simulink model "HVDC_VSC_1CPUcore_dcpl"  (Simulink 8.4)
settings: Solver=ode3  SolverMode=SingleTasking  StartTime=0.0  StopTime=70.0  FixedStep=Ts_Power  RelTol=1e-3  AbsTol=1e-2
PreLoadFcn:
  | Ts_Power=50e-6; Ts_Control=1*Ts_Power; init_cosim_IA; startup_transients_hvdc_vsc;
PostLoadFcn:
  | Ts_Power=50e-6; Ts_Control=1*Ts_Power; init_cosim_IA; startup_transients_hvdc_vsc;
InitFcn:
  | Ts_Power=50e-6; Ts_Control=1*Ts_Power; init_cosim_IA; startup_transients_hvdc_vsc;
values from neighbouring files (symbols this model uses):
  dPref1_2 = 0.125    [startup_transients_hvdc_vsc.m]
  dPref1_2_rlimit = 0.6    [startup_transients_hvdc_vsc.m]
  t_deblock_Pref1 = 0.5    [startup_transients_hvdc_vsc.m]
  t_deblock_Udref2 = 0.3    [startup_transients_hvdc_vsc.m]
  t_dPref1_2 = 25.0    (= 25)    [startup_transients_hvdc_vsc.m]
  t_SwitchITMIdc = 0.2    [startup_transients_hvdc_vsc.m]
  t_SwitchITMVdc = 0.1    [startup_transients_hvdc_vsc.m]
undefined symbols (not defined in the file or in its folder): CLARK, D1, Delta, gcbh, h, intfDelay, level, lib_mesures, magnitude, ResistanceM, rte_drive_private_lib, rte_tsb3level_hiz_rect_cb, sps_rtmsupport, Ts_intf, TSB3_hiZR
libraries: powerlib x183, spsVIMeasurementModel x102, powerlib_extras x71, powerlib_meascontrol x50, rteventslib x26, op_dpl_lib x20, rtlab x12, sps_avr x6, artemis x1
(part 9 of 13)

== system HVDC_VSC_1CPUcore_dcpl/SM_HVDC_VSC/VSC Controller (Station 1)/3-level firing pulse unit for TSB/Subsystem2 ==
  in : Inport
  c+ : Inport  Port=2
  c- : Inport  Port=3
  RTE Logical Operator : rteventslib/Math Operations/RTE Logical Operator  LogicalOperator=NOT  NbrInput=1  NbrMaxEvents=1
  RTE Logical Operator1 : rteventslib/Math Operations/RTE Logical Operator  LogicalOperator=NOT  NbrInput=1  NbrMaxEvents=1
  RTE Relational Operator2 : rteventslib/Math Operations/RTE Relational Operator  RelationalOperator=>=  NumberMaxEvents=1  SampleTime=Ts
  RTE Relational Operator3 : rteventslib/Math Operations/RTE Relational Operator  RelationalOperator=<=  NumberMaxEvents=1  SampleTime=Ts
  1 : Outport
  2 : Outport  Port=2
  3 : Outport  Port=3
  4 : Outport  Port=4
  wires:
  RTE Logical Operator/1 -> 3/1
  RTE Logical Operator1/1 -> 2/1
  RTE Relational Operator3/1 -> 4/1, RTE Logical Operator1/1
  RTE Relational Operator2/1 -> 1/1, RTE Logical Operator/1
  c-/1 -> RTE Relational Operator3/2
  c+/1 -> RTE Relational Operator2/2
  in/1 -> RTE Relational Operator2/1, RTE Relational Operator3/1

== system HVDC_VSC_1CPUcore_dcpl/SM_HVDC_VSC/VSC Controller (Station 1)/3-level firing pulse unit for TSB/Subsystem6 ==
  in : Inport
  c+ : Inport  Port=2
  c- : Inport  Port=3
  RTE Logical Operator : rteventslib/Math Operations/RTE Logical Operator  LogicalOperator=NOT  NbrInput=1  NbrMaxEvents=1
  RTE Logical Operator1 : rteventslib/Math Operations/RTE Logical Operator  LogicalOperator=NOT  NbrInput=1  NbrMaxEvents=1
  RTE Relational Operator2 : rteventslib/Math Operations/RTE Relational Operator  RelationalOperator=>=  NumberMaxEvents=1  SampleTime=Ts
  RTE Relational Operator3 : rteventslib/Math Operations/RTE Relational Operator  RelationalOperator=<=  NumberMaxEvents=1  SampleTime=Ts
  1 : Outport
  2 : Outport  Port=2
  3 : Outport  Port=3
  4 : Outport  Port=4
  wires:
  RTE Logical Operator/1 -> 3/1
  RTE Logical Operator1/1 -> 2/1
  RTE Relational Operator3/1 -> 4/1, RTE Logical Operator1/1
  RTE Relational Operator2/1 -> 1/1, RTE Logical Operator/1
  c-/1 -> RTE Relational Operator3/2
  c+/1 -> RTE Relational Operator2/2
  in/1 -> RTE Relational Operator2/1, RTE Relational Operator3/1

== system HVDC_VSC_1CPUcore_dcpl/SM_HVDC_VSC/VSC Controller (Station 1)/Discrete VSC Controller (Station 1)/Clark Transformations ==
  note: 0: Y-Y
      | 1: Y-D1
      | 2: Y-D11
  note: Clark's Transformations
  "U_abc " : Inport
  "I_abc " : Inport  Port=2
  "Uf_abc " : Inport  Port=3
  "Iv_abc " : Inport  Port=4
  "CLARK " : Subsystem  AncestorBlock=lib_mesures/CLARK
  "CLARK  " : Subsystem  AncestorBlock=lib_mesures/CLARK
  CLARK_YD : Subsystem
  "CLARK_YD " : Subsystem
  Constant2 : Constant  Value=Tr_connection
  Selector{,1..3} (4 alike) : Selector  InputPortWidth=3  Indices=[1 2]
  U_AB : Outport
  I_AB : Outport  Port=2
  Uf_AB : Outport  Port=3
  Iv_AB : Outport  Port=4
  wires:
  Constant2/1 -> "CLARK_YD "/2(Tr_conx), CLARK_YD/2(Tr_conx)
  "U_abc "/1 -> CLARK_YD/1(abc)
  "I_abc "/1 -> "CLARK_YD "/1(abc)
  "Uf_abc "/1 -> "CLARK "/1(abc)
  "Iv_abc "/1 -> "CLARK  "/1(abc)
  CLARK_YD/1(AB0) -> Selector/1
  "CLARK "/1(AB0) -> Selector2/1
  "CLARK  "/1(AB0) -> Selector3/1
  "CLARK_YD "/1(AB0) -> Selector1/1
  Selector/1 -> U_AB/1
  Selector1/1 -> I_AB/1
  Selector2/1 -> Uf_AB/1
  Selector3/1 -> Iv_AB/1

== system HVDC_VSC_1CPUcore_dcpl/SM_HVDC_VSC/VSC Controller (Station 1)/Discrete VSC Controller (Station 1)/DC Voltage Balance Control ==
  note: DC Voltage Balance Control
  Vref_lim_abc : Inport
  Iv_abc : Inport  Port=2
  Udc_pn : Inport  Port=3
  Freq : Inport  Port=4
  activate_reg : Inport  Port=5
  Constant8 : Constant  Value=0
  First-Order_LP f0_dcvbc : powerlib_extras/Discrete  Control Blocks/Discrete 1st-Order Filter  FilterType=Lowpass  Tc=1/(2*pi*f0_dcvbc)  Ts=Ts_Control  Initialize=off  Vac_Init=[0.8 -25 60]  Vdc_Init=-0.4  PlotResponse=off  param1=[1 500 0.1]
  Gain4 : Gain  Gain=k_pu2nom_Vdc  SaturateOnIntegerOverflow=on  OutDataTypeStr=Inherit: Same as input  ParamDataTypeStr=Inherit: Same as input
  Regulator : Subsystem  TreatAsAtomicUnit=on
  Sum : Sum  Inputs=1  SaturateOnIntegerOverflow=on
  Switch2 : Switch  Threshold=0.5  SaturateOnIntegerOverflow=on
  Variable Frequency Mean value : powerlib_extras/Discrete Measurements/Discrete Variable Frequency Mean value  Finit=60  Fmin=f_min_pll  Vinit=0  Ts=Ts_Control
  dVref_abc : Outport
  Udc_0_mean : Outport  Port=2
  wires:
  First-Order_LP f0_dcvbc/1 -> Variable Frequency Mean value/2
  Sum/1 -> First-Order_LP f0_dcvbc/1
  Vref_lim_abc/1 -> Regulator/1(V_ref_lim_abc)
  Iv_abc/1 -> Regulator/2(Iv_abc)
  Udc_pn/1 -> Sum/1
  Freq/1 -> Variable Frequency Mean value/1
  Variable Frequency Mean value/1 -> Gain4/1
  Gain4/1 -> Regulator/3(Udc_0_mean), Udc_0_mean/1
  Regulator/1(dV_ref_abc_dcvbc) -> Switch2/1
  Switch2/1 -> dVref_abc/1
  Constant8/1 -> Switch2/3
  activate_reg/1 -> Regulator/Enable, Switch2/2

== system HVDC_VSC_1CPUcore_dcpl/SM_HVDC_VSC/VSC Controller (Station 1)/Discrete VSC Controller (Station 1)/Inner Current Loop ==
  note: Inner Current Loop
  U_dq : Inport
  Iv_dq : Inport  Port=2
  Udc_meas : Inport  Port=3
  Iref_dq : Inport  Port=4
  Freq : Inport  Port=5
  sin_cos : Inport  Port=6
  AC_Current_Control : Subsystem
  Constant1 : Constant  Value=0
  Inverse_Clark : Subsystem  AncestorBlock=lib_mesures/CLARK
  Max=10 Min=0 : Saturate  UpperLimit=10  LowerLimit=0
  Mux1 : Mux  Inputs=[2 1]
  Reference_Voltage_Conditioning : Subsystem
  Reference_Voltage_Limitation : Subsystem
  Selector : Selector  InputPortWidth=3  Indices=[ 1 2]
  Variable Frequency Mean value IC:1.0 : powerlib_extras/Discrete Measurements/Discrete Variable Frequency Mean value  Finit=60  Fmin=f_min_pll  Vinit=1.0  Ts=Ts_Control
  dq0 to abo : Subsystem  AncestorBlock=lib_mesures/CLARK
  Vref_lim_abc : Outport
  Vref_lim_AB : Outport  Port=2
  wires:
  Selector/1 -> Vref_lim_AB/1
  Reference_Voltage_Limitation/1(Vref_lim_dq) -> Mux1/1
  Inverse_Clark/1(abc) -> Vref_lim_abc/1
  Mux1/1 -> dq0 to abo/1(dq0)
  Constant1/1 -> Mux1/2
  sin_cos/1 -> dq0 to abo/2(sin_cos)
  dq0 to abo/1(ab0) -> Selector/1, Inverse_Clark/1(AB0)
  Udc_meas/1 -> Variable Frequency Mean value IC:1.0/2
  Variable Frequency Mean value IC:1.0/1 -> Max=10 Min=0/1
  Freq/1 -> Variable Frequency Mean value IC:1.0/1, AC_Current_Control/4(Freq)
  Iref_dq/1 -> AC_Current_Control/2(Iref_dq)
  U_dq/1 -> AC_Current_Control/3(U_dq)
  Reference_Voltage_Conditioning/1(Vref_dq) -> Reference_Voltage_Limitation/1(Vref_dq)
  AC_Current_Control/1(Vref_dq_tmp) -> Reference_Voltage_Conditioning/1(Vref_dq_tmp)
  Max=10 Min=0/1 -> Reference_Voltage_Conditioning/2(Udc_meas_mean)
  Iv_dq/1 -> AC_Current_Control/1(Iv_dq)

== system HVDC_VSC_1CPUcore_dcpl/SM_HVDC_VSC/VSC Controller (Station 1)/Discrete VSC Controller (Station 1)/Outer Active-Reactive Power and Voltage Loop ==
  note: Outer Active-Reactive Power and Voltage Loop
  Udc_meas : Inport
  Uf_meas : Inport  Port=2
  P_meas : Inport  Port=3
  Q_meas : Inport  Port=4
  U_meas : Inport  Port=5
  Pref : Inport  Port=6
  dPref : Inport  Port=7
  Qref : Inport  Port=8
  Udref : Inport  Port=9
  block_status : Inport  Port=10
  Active_Power_Control : Subsystem
  Constant19 : Constant  Value=Ki_dcvc
  Constant20 : Constant  Value=Kp_dcvc
  Constant9 : Constant  Value=P_control
  Current_Reference_Calculation : Subsystem
  Current_Reference_Limitation : Subsystem
  DC_Voltage_Control : Subsystem  TreatAsAtomicUnit=on
  Logical Operator1 : Logic  AllPortsSameDT=off
  Logical Operator4 : Logic  Operator=NOT  AllPortsSameDT=off
  Logical Operator6 : Logic  AllPortsSameDT=off
  Logical Operator7 : Logic  Operator=NOT  AllPortsSameDT=off
  Reactive_Power_Control : Subsystem
  Switch2 : Switch  Threshold=0.5  SaturateOnIntegerOverflow=on
  Iref_dq : Outport
  Pref_ramped : Outport  Port=2
  wires:
  Current_Reference_Limitation/1(Iref_dq) -> Iref_dq/1
  Switch2/1 -> Current_Reference_Limitation/1(Iref_d_tmp)
  Logical Operator4/1 -> Logical Operator1/1, Logical Operator6/2, Active_Power_Control/2(enable_ramp), Reactive_Power_Control/1(enable_control)
  Current_Reference_Calculation/1(Iref_d_crc) -> Switch2/1
  Constant20/1 -> DC_Voltage_Control/4(Kp_dcvc)
  Constant19/1 -> DC_Voltage_Control/3(Ki_dcvc)
  Q_meas/1 -> Reactive_Power_Control/3(Q_meas)
  P_meas/1 -> Active_Power_Control/5(P_meas)
  DC_Voltage_Control/1(Iref_d_dcvc) -> Switch2/3
  Udc_meas/1 -> Active_Power_Control/7(Udc_meas), DC_Voltage_Control/2(Udc_meas)
  block_status/1 -> Logical Operator4/1
  Constant9/1 -> Logical Operator6/1, Current_Reference_Limitation/3(P_control), Logical Operator7/1
  Logical Operator6/1 -> Switch2/2, Active_Power_Control/1(enable_control)
  U_meas/1 -> Reactive_Power_Control/4(U_meas), Active_Power_Control/6(U_meas)
  Current_Reference_Calculation/2(Iref_q_crc) -> Current_Reference_Limitation/2(Iref_q_tmp)
  dPref/1 -> Active_Power_Control/4(dPref)
  Active_Power_Control/1(Pref_apc) -> Current_Reference_Calculation/1(Pref_apc)
  Reactive_Power_Control/1(Qref_rpc) -> Current_Reference_Calculation/2(Qref_rpc)
  Pref/1 -> Active_Power_Control/3(Pref)
  Uf_meas/1 -> Current_Reference_Calculation/3(Uf_meas)
  Qref/1 -> Reactive_Power_Control/2(Qref)
  Logical Operator7/1 -> Logical Operator1/2
  Logical Operator1/1 -> DC_Voltage_Control/Enable
  Udref/1 -> DC_Voltage_Control/1(Udref)
  Active_Power_Control/2(Pref_ramped) -> Pref_ramped/1

== system HVDC_VSC_1CPUcore_dcpl/SM_HVDC_VSC/VSC Controller (Station 1)/Discrete VSC Controller (Station 1)/PLL ==
  note: Discrete 3-phase PLL
  note: Pierre Giroux, Gilbert Sybille
      | Power System Laboratory, IREQ
      | Hydro-Quebec
  U_AB : Inport
  Constant1 : Constant  Value=0
  Constant4 : Constant  Value=2*pi
  Discrete PI Controller : powerlib_extras/Discrete  Control Blocks/Discrete PI Controller  Kp=Kp  Ki=Ki  Par_Limits=2*pi*Finit*[1.25 0.75]  Init=2*pi*Finit  Ts=Ts
  Discrete Rate Limiter : powerlib_extras/Discrete  Control Blocks/Discrete Rate Limiter  R=12  F=-12  Vinit=Finit  Ts=Ts
  Discrete Variable Frequency Mean value : powerlib_extras/Discrete Measurements/Discrete Variable Frequency Mean value  Finit=Finit  Fmin=Fmin  Vinit=0  Ts=Ts
  Discrete  2nd-Order Filter : powerlib_extras/Discrete  Control Blocks/Discrete  2nd-Order Filter  FilterType=Lowpass  Fo=30  Zeta=0.707  Ts=Ts  Initialize=on  Vac_Init=[0 0 Finit]  Vdc_Init=Finit  PlotResponse=off  param1=[1 500 0.1]
  Discrete-Time Integrator : DiscreteIntegrator  InitialCondition=Phase_Init*pi/180  SampleTime=Ts
  Gain10 : Gain  Gain=1/2/pi  SaturateOnIntegerOverflow=on  OutDataTypeStr=Inherit: Same as input  ParamDataTypeStr=Inherit: Same as input
  Math Function : Math  Operator=mod  SaturateOnIntegerOverflow=on
  Mux1 : Mux  Inputs=[2 1]
  Mux2 : Mux  Inputs=2
  Selector : Selector  InputPortWidth=3  Indices=2
  Trigonometric Function : Trigonometry
  Trigonometric Function2 : Trigonometry  Operator=cos
  Unit Delay : UnitDelay  InitialCondition=Finit  SampleTime=Ts
  "ab0->dq0 " : Subsystem  AncestorBlock=lib_mesures/CLARK
  Freq : Outport
  theta : Outport  Port=2
  Sin_Cos : Outport  Port=3
  wires:
  Constant1/1 -> Mux1/2
  Mux1/1 -> "ab0->dq0 "/1(ab0)
  U_AB/1 -> Mux1/1
  Discrete Variable Frequency Mean value/1 -> Discrete PI Controller/1
  "ab0->dq0 "/1(dq0) -> Selector/1
  Constant4/1 -> Math Function/2
  Discrete-Time Integrator/1 -> Math Function/1
  Math Function/1 -> Trigonometric Function/1, Trigonometric Function2/1, theta/1
  Trigonometric Function/1 -> Mux2/1
  Trigonometric Function2/1 -> Mux2/2
  Mux2/1 -> "ab0->dq0 "/2(sin_cos), Sin_Cos/1
  Discrete PI Controller/1 -> Discrete-Time Integrator/1, Gain10/1  "W"
  Gain10/1 -> Discrete Rate Limiter/1
  Discrete Rate Limiter/1 -> Discrete  2nd-Order Filter/1
  Unit Delay/1 -> Freq/1, Discrete Variable Frequency Mean value/1
  Discrete  2nd-Order Filter/1 -> Unit Delay/1
  Selector/1 -> Discrete Variable Frequency Mean value/2  "Vq"

== system HVDC_VSC_1CPUcore_dcpl/SM_HVDC_VSC/VSC Controller (Station 1)/Discrete VSC Controller (Station 1)/Signal Calculations ==
  U_AB : Inport
  I_AB : Inport  Port=2
  Uf_AB : Inport  Port=3
  Vref_lim_AB : Inport  Port=4
  Udc_pn : Inport  Port=5
  Idc_pn : Inport  Port=6
  Freq : Inport  Port=7
  2nd-Order Filter : powerlib_extras/Discrete  Control Blocks/Discrete  2nd-Order Filter  FilterType=Lowpass  Fo=f0_sc  Zeta=zeta_sc  Ts=Ts_Control  Initialize=off  Vac_Init=[0.8 -25 60]  Vdc_Init=-0.4  PlotResponse=off  param1=[1 500 1]
  2nd-Order Filter2 : powerlib_extras/Discrete  Control Blocks/Discrete  2nd-Order Filter  FilterType=Lowpass  Fo=f0_sc  Zeta=zeta_sc  Ts=Ts_Control  Initialize=off  Vac_Init=[0.8 -25 60]  Vdc_Init=-0.4  PlotResponse=off  param1=[1 500 1]
  "2nd-Order Filter " : powerlib_extras/Discrete  Control Blocks/Discrete  2nd-Order Filter  FilterType=Lowpass  Fo=f0_sc  Zeta=zeta_sc  Ts=Ts_Control  Initialize=off  Vac_Init=[0.8 -25 60]  Vdc_Init=-0.4  PlotResponse=off  param1=[1 500 1]
  "2nd-Order Filter  " : powerlib_extras/Discrete  Control Blocks/Discrete  2nd-Order Filter  FilterType=Lowpass  Fo=f0_sc  Zeta=zeta_sc  Ts=Ts_Control  Initialize=off  Vac_Init=[0.8 -25 60]  Vdc_Init=-0.4  PlotResponse=off  param1=[1 500 1]
  2nd-Order Filter 1\ : powerlib_extras/Discrete  Control Blocks/Discrete  2nd-Order Filter  FilterType=Lowpass  Fo=f0_sc  Zeta=zeta_sc  Ts=Ts_Control  Initialize=off  Vac_Init=[0.8 -25 60]  Vdc_Init=-0.4  PlotResponse=off  param1=[1 500 1]
  Active_Power : Subsystem
  DC_Current : Subsystem
  DC_Voltage : Subsystem
  Demux : Demux  Outputs=2
  Demux1 : Demux  Outputs=2
  Filter_Bus_Voltage : Subsystem
  Gain1 : Gain  Gain=k_pu2nom_Vdc*k_pu2nom_Idc  SaturateOnIntegerOverflow=on  OutDataTypeStr=Inherit: Same as input  ParamDataTypeStr=Inherit: Same as input
  Modulation_Index : Subsystem
  PCC_Voltage : Subsystem
  Product5 : Product  SaturateOnIntegerOverflow=on  OutDataTypeStr=Inherit: Same as first input
  Reactive_Power : Subsystem
  Variable Frequency Mean value IC: 0 : powerlib_extras/Discrete Measurements/Discrete Variable Frequency Mean value  Finit=60  Fmin=f_min_pll  Vinit=0  Ts=Ts_Control
  Pdc_meas : Outport
  Mod_index : Outport  Port=2
  Udc_meas : Outport  Port=3
  Uf_meas : Outport  Port=4
  P_meas : Outport  Port=5
  Q_meas : Outport  Port=6
  U_meas : Outport  Port=7
  wires:
  Gain1/1 -> Pdc_meas/1
  Freq/1 -> Variable Frequency Mean value IC: 0/1
  Product5/1 -> Gain1/1
  Variable Frequency Mean value IC: 0/1 -> Product5/2
  2nd-Order Filter 1\/1 -> Uf_meas/1
  "2nd-Order Filter "/1 -> Mod_index/1
  Filter_Bus_Voltage/1(Uf_meas) -> 2nd-Order Filter 1\/1
  PCC_Voltage/1(Upcc) -> "2nd-Order Filter  "/1
  "2nd-Order Filter  "/1 -> U_meas/1
  Active_Power/1(Ppcc) -> 2nd-Order Filter/1
  2nd-Order Filter/1 -> P_meas/1
  Reactive_Power/1(Qpcc) -> 2nd-Order Filter2/1
  2nd-Order Filter2/1 -> Q_meas/1
  Modulation_Index/1(Mod_index) -> "2nd-Order Filter "/1
  Demux/2 -> DC_Voltage/2(Udc_n)
  Uf_AB/1 -> Filter_Bus_Voltage/1(Uf_AB)
  U_AB/1 -> PCC_Voltage/1(U_AB), Active_Power/1(U_AB), Reactive_Power/1(U_AB)
  I_AB/1 -> Active_Power/2(I_AB), Reactive_Power/2(I_AB)
  DC_Voltage/1(Udc_meas) -> Product5/1, Udc_meas/1, Modulation_Index/2(Udc_meas)
  DC_Current/1(Idc_meas) -> Variable Frequency Mean value IC: 0/2
  Udc_pn/1 -> Demux/1
  Demux/1 -> DC_Voltage/1(Udc_p)
  Demux1/1 -> DC_Current/1(Idc_p)
  Demux1/2 -> DC_Current/2(Idc_n)
  Idc_pn/1 -> Demux1/1
  Vref_lim_AB/1 -> Modulation_Index/1(Vref_lim_AB)

== system HVDC_VSC_1CPUcore_dcpl/SM_HVDC_VSC/VSC Controller (Station 1)/Discrete VSC Controller (Station 1)/dq  Transformations ==
  note: dq Transformations
  U_AB : Inport
  Iv_AB : Inport  Port=2
  sin_cos : Inport  Port=3
  Constant1 : Constant  Value=0
  Mux1 : Mux  Inputs=[2 1]
  Mux4 : Mux  Inputs=[2 1]
  Selector : Selector  InputPortWidth=3  Indices=[1 2]
  Selector3 : Selector  InputPortWidth=3  Indices=[1 2]
  ab0_to_dq0 : Subsystem  AncestorBlock=lib_mesures/CLARK
  "ab0_to_dq0   " : Subsystem  AncestorBlock=lib_mesures/CLARK
  U_dq : Outport
  Iv_dq : Outport  Port=2
  wires:
  Constant1/1 -> Mux4/2, Mux1/2
  Mux4/1 -> "ab0_to_dq0   "/1(ab0)
  Iv_AB/1 -> Mux4/1
  Mux1/1 -> ab0_to_dq0/1(ab0)
  U_AB/1 -> Mux1/1
  "ab0_to_dq0   "/1(dq0) -> Selector3/1
  ab0_to_dq0/1(dq0) -> Selector/1
  sin_cos/1 -> "ab0_to_dq0   "/2(sin_cos), ab0_to_dq0/2(sin_cos)
  Selector/1 -> U_dq/1
  Selector3/1 -> Iv_dq/1

== system HVDC_VSC_1CPUcore_dcpl/SM_HVDC_VSC/VSC Controller (Station 2)/3-level firing pulse unit for TSB/Carriers Generator ==
  theta : Inport
  Constant2 : Constant  Value=0.5
  Gain1 : Gain  Gain=1/pi  SaturateOnIntegerOverflow=on  OutDataTypeStr=Inherit: Same as input  ParamDataTypeStr=Inherit: Same as input
  Sum1 : Sum  SaturateOnIntegerOverflow=on  InputSameDT=on  OutDataTypeStr=Inherit: Same as first input
  Sum2 : Sum  Inputs=+-  SaturateOnIntegerOverflow=on  InputSameDT=on  OutDataTypeStr=Inherit: Same as first input
  Trigonometric Function : Trigonometry  Operator=asin
  Trigonometric Function3 : Trigonometry
  C+ : Outport
  C- : Outport  Port=2
  wires:
  Trigonometric Function/1 -> Gain1/1
  Trigonometric Function3/1 -> Trigonometric Function/1
  Gain1/1 -> Sum1/1, Sum2/1
  Constant2/1 -> Sum2/2, Sum1/2
  Sum2/1 -> C-/1  "Carrier 1-"
  Sum1/1 -> C+/1  "Carrier 1+"
  theta/1 -> Trigonometric Function3/1

== system HVDC_VSC_1CPUcore_dcpl/SM_HVDC_VSC/VSC Controller (Station 2)/3-level firing pulse unit for TSB/Subsystem1 ==
  in : Inport
  c+ : Inport  Port=2
  c- : Inport  Port=3
  RTE Logical Operator : rteventslib/Math Operations/RTE Logical Operator  LogicalOperator=NOT  NbrInput=1  NbrMaxEvents=1
  RTE Logical Operator1 : rteventslib/Math Operations/RTE Logical Operator  LogicalOperator=NOT  NbrInput=1  NbrMaxEvents=1
  RTE Relational Operator2 : rteventslib/Math Operations/RTE Relational Operator  RelationalOperator=>=  NumberMaxEvents=1  SampleTime=Ts
  RTE Relational Operator3 : rteventslib/Math Operations/RTE Relational Operator  RelationalOperator=<=  NumberMaxEvents=1  SampleTime=Ts
  1 : Outport
  2 : Outport  Port=2
  3 : Outport  Port=3
  4 : Outport  Port=4
  wires:
  in/1 -> RTE Relational Operator3/1, RTE Relational Operator2/1
  c+/1 -> RTE Relational Operator2/2
  c-/1 -> RTE Relational Operator3/2
  RTE Relational Operator2/1 -> RTE Logical Operator/1, 1/1
  RTE Relational Operator3/1 -> RTE Logical Operator1/1, 4/1
  RTE Logical Operator1/1 -> 2/1
  RTE Logical Operator/1 -> 3/1

== system HVDC_VSC_1CPUcore_dcpl/SM_HVDC_VSC/VSC Controller (Station 2)/3-level firing pulse unit for TSB/Subsystem2 ==
  in : Inport
  c+ : Inport  Port=2
  c- : Inport  Port=3
  RTE Logical Operator : rteventslib/Math Operations/RTE Logical Operator  LogicalOperator=NOT  NbrInput=1  NbrMaxEvents=1
  RTE Logical Operator1 : rteventslib/Math Operations/RTE Logical Operator  LogicalOperator=NOT  NbrInput=1  NbrMaxEvents=1
  RTE Relational Operator2 : rteventslib/Math Operations/RTE Relational Operator  RelationalOperator=>=  NumberMaxEvents=1  SampleTime=Ts
  RTE Relational Operator3 : rteventslib/Math Operations/RTE Relational Operator  RelationalOperator=<=  NumberMaxEvents=1  SampleTime=Ts
  1 : Outport
  2 : Outport  Port=2
  3 : Outport  Port=3
  4 : Outport  Port=4
  wires:
  RTE Logical Operator/1 -> 3/1
  RTE Logical Operator1/1 -> 2/1
  RTE Relational Operator3/1 -> 4/1, RTE Logical Operator1/1
  RTE Relational Operator2/1 -> 1/1, RTE Logical Operator/1
  c-/1 -> RTE Relational Operator3/2
  c+/1 -> RTE Relational Operator2/2
  in/1 -> RTE Relational Operator2/1, RTE Relational Operator3/1

== system HVDC_VSC_1CPUcore_dcpl/SM_HVDC_VSC/VSC Controller (Station 2)/3-level firing pulse unit for TSB/Subsystem6 ==
  in : Inport
  c+ : Inport  Port=2
  c- : Inport  Port=3
  RTE Logical Operator : rteventslib/Math Operations/RTE Logical Operator  LogicalOperator=NOT  NbrInput=1  NbrMaxEvents=1
  RTE Logical Operator1 : rteventslib/Math Operations/RTE Logical Operator  LogicalOperator=NOT  NbrInput=1  NbrMaxEvents=1
  RTE Relational Operator2 : rteventslib/Math Operations/RTE Relational Operator  RelationalOperator=>=  NumberMaxEvents=1  SampleTime=Ts
  RTE Relational Operator3 : rteventslib/Math Operations/RTE Relational Operator  RelationalOperator=<=  NumberMaxEvents=1  SampleTime=Ts
  1 : Outport
  2 : Outport  Port=2
  3 : Outport  Port=3
  4 : Outport  Port=4
  wires:
  RTE Logical Operator/1 -> 3/1
  RTE Logical Operator1/1 -> 2/1
  RTE Relational Operator3/1 -> 4/1, RTE Logical Operator1/1
  RTE Relational Operator2/1 -> 1/1, RTE Logical Operator/1
  c-/1 -> RTE Relational Operator3/2
  c+/1 -> RTE Relational Operator2/2
  in/1 -> RTE Relational Operator2/1, RTE Relational Operator3/1

== system HVDC_VSC_1CPUcore_dcpl/SM_HVDC_VSC/VSC Controller (Station 2)/Discrete VSC Controller (Station 2)/Clark Transformations ==
  note: 0: Y-Y
      | 1: Y-D1
      | 2: Y-D11
  note: Clark's Transformations
  "U_abc " : Inport
  "I_abc " : Inport  Port=2
  "Uf_abc " : Inport  Port=3
  "Iv_abc " : Inport  Port=4
  "CLARK " : Subsystem  AncestorBlock=lib_mesures/CLARK
  "CLARK  " : Subsystem  AncestorBlock=lib_mesures/CLARK
  CLARK_YD : Subsystem
  "CLARK_YD " : Subsystem
  Constant2 : Constant  Value=Tr_connection
  Selector{,1..3} (4 alike) : Selector  InputPortWidth=3  Indices=[1 2]
  U_AB : Outport
  I_AB : Outport  Port=2
  Uf_AB : Outport  Port=3
  Iv_AB : Outport  Port=4
  wires:
  Constant2/1 -> "CLARK_YD "/2(Tr_conx), CLARK_YD/2(Tr_conx)
  "U_abc "/1 -> CLARK_YD/1(abc)
  "I_abc "/1 -> "CLARK_YD "/1(abc)
  "Uf_abc "/1 -> "CLARK "/1(abc)
  "Iv_abc "/1 -> "CLARK  "/1(abc)
  CLARK_YD/1(AB0) -> Selector/1
  "CLARK "/1(AB0) -> Selector2/1
  "CLARK  "/1(AB0) -> Selector3/1
  "CLARK_YD "/1(AB0) -> Selector1/1
  Selector/1 -> U_AB/1
  Selector1/1 -> I_AB/1
  Selector2/1 -> Uf_AB/1
  Selector3/1 -> Iv_AB/1

== system HVDC_VSC_1CPUcore_dcpl/SM_HVDC_VSC/VSC Controller (Station 2)/Discrete VSC Controller (Station 2)/DC Voltage Balance Control ==
  note: DC Voltage Balance Control
  Vref_lim_abc : Inport
  Iv_abc : Inport  Port=2
  Udc_pn : Inport  Port=3
  Freq : Inport  Port=4
  activate_reg : Inport  Port=5
  Constant8 : Constant  Value=0
  First-Order_LP f0_dcvbc : powerlib_extras/Discrete  Control Blocks/Discrete 1st-Order Filter  FilterType=Lowpass  Tc=1/(2*pi*f0_dcvbc)  Ts=Ts_Control  Initialize=off  Vac_Init=[0.8 -25 60]  Vdc_Init=-0.4  PlotResponse=off  param1=[1 500 0.1]
  Gain4 : Gain  Gain=k_pu2nom_Vdc  SaturateOnIntegerOverflow=on  OutDataTypeStr=Inherit: Same as input  ParamDataTypeStr=Inherit: Same as input
  Regulator : Subsystem  TreatAsAtomicUnit=on
  Sum : Sum  Inputs=1  SaturateOnIntegerOverflow=on
  Switch2 : Switch  Threshold=0.5  SaturateOnIntegerOverflow=on
  Variable Frequency Mean value : powerlib_extras/Discrete Measurements/Discrete Variable Frequency Mean value  Finit=50  Fmin=f_min_pll  Vinit=0  Ts=Ts_Control
  dVref_abc : Outport
  Udc_0_mean : Outport  Port=2
  wires:
  First-Order_LP f0_dcvbc/1 -> Variable Frequency Mean value/2
  Sum/1 -> First-Order_LP f0_dcvbc/1
  Vref_lim_abc/1 -> Regulator/1(V_ref_lim_abc)
  Iv_abc/1 -> Regulator/2(Iv_abc)
  Udc_pn/1 -> Sum/1
  Freq/1 -> Variable Frequency Mean value/1
  Variable Frequency Mean value/1 -> Gain4/1
  Gain4/1 -> Regulator/3(Udc_0_mean), Udc_0_mean/1
  Regulator/1(dV_ref_abc_dcvbc) -> Switch2/1
  Switch2/1 -> dVref_abc/1
  Constant8/1 -> Switch2/3
  activate_reg/1 -> Regulator/Enable, Switch2/2

== system HVDC_VSC_1CPUcore_dcpl/SM_HVDC_VSC/VSC Controller (Station 2)/Discrete VSC Controller (Station 2)/Inner Current Loop ==
  note: Inner Current Loop
  U_dq : Inport
  Iv_dq : Inport  Port=2
  Udc_meas : Inport  Port=3
  Iref_dq : Inport  Port=4
  Freq : Inport  Port=5
  sin_cos : Inport  Port=6
  AC_Current_Control : Subsystem
  Constant1 : Constant  Value=0
  Inverse_Clark : Subsystem  AncestorBlock=lib_mesures/CLARK
  Max=10 Min=0 : Saturate  UpperLimit=10  LowerLimit=0
  Mux1 : Mux  Inputs=[2 1]
  Reference_Voltage_Conditioning : Subsystem
  Reference_Voltage_Limitation : Subsystem
  Selector : Selector  InputPortWidth=3  Indices=[ 1 2]
  Variable Frequency Mean value IC:1.0 : powerlib_extras/Discrete Measurements/Discrete Variable Frequency Mean value  Finit=50  Fmin=f_min_pll  Vinit=1.0  Ts=Ts_Control
  dq0 to abo : Subsystem  AncestorBlock=lib_mesures/CLARK
  Vref_lim_abc : Outport
  Vref_lim_AB : Outport  Port=2
  wires:
  Selector/1 -> Vref_lim_AB/1
  Reference_Voltage_Limitation/1(Vref_lim_dq) -> Mux1/1
  Inverse_Clark/1(abc) -> Vref_lim_abc/1
  Mux1/1 -> dq0 to abo/1(dq0)
  Constant1/1 -> Mux1/2
  sin_cos/1 -> dq0 to abo/2(sin_cos)
  dq0 to abo/1(ab0) -> Selector/1, Inverse_Clark/1(AB0)
  Udc_meas/1 -> Variable Frequency Mean value IC:1.0/2
  Variable Frequency Mean value IC:1.0/1 -> Max=10 Min=0/1
  Freq/1 -> Variable Frequency Mean value IC:1.0/1, AC_Current_Control/4(Freq)
  Iref_dq/1 -> AC_Current_Control/2(Iref_dq)
  U_dq/1 -> AC_Current_Control/3(U_dq)
  Reference_Voltage_Conditioning/1(Vref_dq) -> Reference_Voltage_Limitation/1(Vref_dq)
  AC_Current_Control/1(Vref_dq_tmp) -> Reference_Voltage_Conditioning/1(Vref_dq_tmp)
  Max=10 Min=0/1 -> Reference_Voltage_Conditioning/2(Udc_meas_mean)
  Iv_dq/1 -> AC_Current_Control/1(Iv_dq)

== system HVDC_VSC_1CPUcore_dcpl/SM_HVDC_VSC/VSC Controller (Station 2)/Discrete VSC Controller (Station 2)/Outer Active-Reactive Power and Voltage Loop ==
  note: Outer Active-Reactive Power and Voltage Loop
  Udc_meas : Inport
  Uf_meas : Inport  Port=2
  P_meas : Inport  Port=3
  Q_meas : Inport  Port=4
  U_meas : Inport  Port=5
  Pref : Inport  Port=6
  dPref : Inport  Port=7
  Qref : Inport  Port=8
  Udref : Inport  Port=9
  block_status : Inport  Port=10
  Active_Power_Control : Subsystem
  Constant19 : Constant  Value=Ki_dcvc
  Constant20 : Constant  Value=Kp_dcvc
  Constant9 : Constant  Value=P_control
  Current_Reference_Calculation : Subsystem
  Current_Reference_Limitation : Subsystem
  DC_Voltage_Control : Subsystem  TreatAsAtomicUnit=on
  Logical Operator1 : Logic  AllPortsSameDT=off
  Logical Operator4 : Logic  Operator=NOT  AllPortsSameDT=off
  Logical Operator6 : Logic  AllPortsSameDT=off
  Logical Operator7 : Logic  Operator=NOT  AllPortsSameDT=off
  Reactive_Power_Control : Subsystem
  Switch2 : Switch  Threshold=0.5  SaturateOnIntegerOverflow=on
  Iref_dq : Outport
  Pref_ramped : Outport  Port=2
  wires:
  Current_Reference_Limitation/1(Iref_dq) -> Iref_dq/1
  Switch2/1 -> Current_Reference_Limitation/1(Iref_d_tmp)
  Logical Operator4/1 -> Logical Operator1/1, Logical Operator6/2, Active_Power_Control/2(enable_ramp), Reactive_Power_Control/1(enable_control)
  Current_Reference_Calculation/1(Iref_d_crc) -> Switch2/1
  Constant20/1 -> DC_Voltage_Control/4(Kp_dcvc)
  Constant19/1 -> DC_Voltage_Control/3(Ki_dcvc)
  Q_meas/1 -> Reactive_Power_Control/3(Q_meas)
  P_meas/1 -> Active_Power_Control/5(P_meas)
  DC_Voltage_Control/1(Iref_d_dcvc) -> Switch2/3
  Udc_meas/1 -> Active_Power_Control/7(Udc_meas), DC_Voltage_Control/2(Udc_meas)
  block_status/1 -> Logical Operator4/1
  Constant9/1 -> Logical Operator6/1, Current_Reference_Limitation/3(P_control), Logical Operator7/1
  Logical Operator6/1 -> Switch2/2, Active_Power_Control/1(enable_control)
  U_meas/1 -> Reactive_Power_Control/4(U_meas), Active_Power_Control/6(U_meas)
  Current_Reference_Calculation/2(Iref_q_crc) -> Current_Reference_Limitation/2(Iref_q_tmp)
  dPref/1 -> Active_Power_Control/4(dPref)
  Active_Power_Control/1(Pref_apc) -> Current_Reference_Calculation/1(Pref_apc)
  Reactive_Power_Control/1(Qref_rpc) -> Current_Reference_Calculation/2(Qref_rpc)
  Pref/1 -> Active_Power_Control/3(Pref)
  Uf_meas/1 -> Current_Reference_Calculation/3(Uf_meas)
  Qref/1 -> Reactive_Power_Control/2(Qref)
  Logical Operator7/1 -> Logical Operator1/2
  Logical Operator1/1 -> DC_Voltage_Control/Enable
  Udref/1 -> DC_Voltage_Control/1(Udref)
  Active_Power_Control/2(Pref_ramped) -> Pref_ramped/1

== system HVDC_VSC_1CPUcore_dcpl/SM_HVDC_VSC/VSC Controller (Station 2)/Discrete VSC Controller (Station 2)/PLL ==
  note: Discrete 3-phase PLL
  note: Pierre Giroux, Gilbert Sybille
      | Power System Laboratory, IREQ
      | Hydro-Quebec
  U_AB : Inport
  Constant1 : Constant  Value=0
  Constant4 : Constant  Value=2*pi
  Discrete PI Controller : powerlib_extras/Discrete  Control Blocks/Discrete PI Controller  Kp=Kp  Ki=Ki  Par_Limits=2*pi*Finit*[1.25 0.75]  Init=2*pi*Finit  Ts=Ts
  Discrete Rate Limiter : powerlib_extras/Discrete  Control Blocks/Discrete Rate Limiter  R=12  F=-12  Vinit=Finit  Ts=Ts
  Discrete Variable Frequency Mean value : powerlib_extras/Discrete Measurements/Discrete Variable Frequency Mean value  Finit=Finit  Fmin=Fmin  Vinit=0  Ts=Ts
  Discrete  2nd-Order Filter : powerlib_extras/Discrete  Control Blocks/Discrete  2nd-Order Filter  FilterType=Lowpass  Fo=25  Zeta=0.707  Ts=Ts  Initialize=on  Vac_Init=[0 0 Finit]  Vdc_Init=Finit  PlotResponse=off  param1=[1 500 0.1]
  Discrete-Time Integrator : DiscreteIntegrator  InitialCondition=Phase_Init*pi/180  SampleTime=Ts
  Gain10 : Gain  Gain=1/2/pi  SaturateOnIntegerOverflow=on  OutDataTypeStr=Inherit: Same as input  ParamDataTypeStr=Inherit: Same as input
  Math Function : Math  Operator=mod  SaturateOnIntegerOverflow=on
  Mux1 : Mux  Inputs=[2 1]
  Mux2 : Mux  Inputs=2
  Selector : Selector  InputPortWidth=3  Indices=2
  Trigonometric Function : Trigonometry
  Trigonometric Function2 : Trigonometry  Operator=cos
  Unit Delay : UnitDelay  InitialCondition=Finit  SampleTime=Ts
  "ab0->dq0 " : Subsystem  AncestorBlock=lib_mesures/CLARK
  Freq : Outport
  theta : Outport  Port=2
  Sin_Cos : Outport  Port=3
  wires:
  Constant1/1 -> Mux1/2
  Mux1/1 -> "ab0->dq0 "/1(ab0)
  U_AB/1 -> Mux1/1
  Discrete Variable Frequency Mean value/1 -> Discrete PI Controller/1
  "ab0->dq0 "/1(dq0) -> Selector/1
  Constant4/1 -> Math Function/2
  Discrete-Time Integrator/1 -> Math Function/1
  Math Function/1 -> Trigonometric Function/1, Trigonometric Function2/1, theta/1
  Trigonometric Function/1 -> Mux2/1
  Trigonometric Function2/1 -> Mux2/2
  Mux2/1 -> "ab0->dq0 "/2(sin_cos), Sin_Cos/1
  Discrete PI Controller/1 -> Discrete-Time Integrator/1, Gain10/1  "W"
  Gain10/1 -> Discrete Rate Limiter/1
  Discrete Rate Limiter/1 -> Discrete  2nd-Order Filter/1
  Unit Delay/1 -> Freq/1, Discrete Variable Frequency Mean value/1
  Discrete  2nd-Order Filter/1 -> Unit Delay/1
  Selector/1 -> Discrete Variable Frequency Mean value/2  "Vq"

== system HVDC_VSC_1CPUcore_dcpl/SM_HVDC_VSC/VSC Controller (Station 2)/Discrete VSC Controller (Station 2)/Signal Calculations ==
  U_AB : Inport
  I_AB : Inport  Port=2
  Uf_AB : Inport  Port=3
  Vref_lim_AB : Inport  Port=4
  Udc_pn : Inport  Port=5
  Idc_pn : Inport  Port=6
  Freq : Inport  Port=7
  2nd-Order Filter : powerlib_extras/Discrete  Control Blocks/Discrete  2nd-Order Filter  FilterType=Lowpass  Fo=f0_sc  Zeta=zeta_sc  Ts=Ts_Control  Initialize=off  Vac_Init=[0.8 -25 60]  Vdc_Init=-0.4  PlotResponse=off  param1=[1 500 1]
  2nd-Order Filter2 : powerlib_extras/Discrete  Control Blocks/Discrete  2nd-Order Filter  FilterType=Lowpass  Fo=f0_sc  Zeta=zeta_sc  Ts=Ts_Control  Initialize=off  Vac_Init=[0.8 -25 60]  Vdc_Init=-0.4  PlotResponse=off  param1=[1 500 1]
  "2nd-Order Filter " : powerlib_extras/Discrete  Control Blocks/Discrete  2nd-Order Filter  FilterType=Lowpass  Fo=f0_sc  Zeta=zeta_sc  Ts=Ts_Control  Initialize=off  Vac_Init=[0.8 -25 60]  Vdc_Init=-0.4  PlotResponse=off  param1=[1 500 1]
  "2nd-Order Filter  " : powerlib_extras/Discrete  Control Blocks/Discrete  2nd-Order Filter  FilterType=Lowpass  Fo=f0_sc  Zeta=zeta_sc  Ts=Ts_Control  Initialize=off  Vac_Init=[0.8 -25 60]  Vdc_Init=-0.4  PlotResponse=off  param1=[1 500 1]
  2nd-Order Filter 1\ : powerlib_extras/Discrete  Control Blocks/Discrete  2nd-Order Filter  FilterType=Lowpass  Fo=f0_sc  Zeta=zeta_sc  Ts=Ts_Control  Initialize=off  Vac_Init=[0.8 -25 60]  Vdc_Init=-0.4  PlotResponse=off  param1=[1 500 1]
  Active_Power : Subsystem
  DC_Current : Subsystem
  DC_Voltage : Subsystem
  Demux : Demux  Outputs=2
  Demux1 : Demux  Outputs=2
  Filter_Bus_Voltage : Subsystem
  Gain1 : Gain  Gain=k_pu2nom_Vdc*k_pu2nom_Idc  SaturateOnIntegerOverflow=on  OutDataTypeStr=Inherit: Same as input  ParamDataTypeStr=Inherit: Same as input
  Modulation_Index : Subsystem
  PCC_Voltage : Subsystem
  Product5 : Product  SaturateOnIntegerOverflow=on  OutDataTypeStr=Inherit: Same as first input
  Reactive_Power : Subsystem
  Variable Frequency Mean value IC: 0 : powerlib_extras/Discrete Measurements/Discrete Variable Frequency Mean value  Finit=50  Fmin=f_min_pll  Vinit=0  Ts=Ts_Control
  Pdc_meas : Outport
  Mod_index : Outport  Port=2
  Udc_meas : Outport  Port=3
  Uf_meas : Outport  Port=4
  P_meas : Outport  Port=5
  Q_meas : Outport  Port=6
  U_meas : Outport  Port=7
  wires:
  Gain1/1 -> Pdc_meas/1
  Freq/1 -> Variable Frequency Mean value IC: 0/1
  Product5/1 -> Gain1/1
  Variable Frequency Mean value IC: 0/1 -> Product5/2
  2nd-Order Filter 1\/1 -> Uf_meas/1
  "2nd-Order Filter "/1 -> Mod_index/1
  Filter_Bus_Voltage/1(Uf_meas) -> 2nd-Order Filter 1\/1
  PCC_Voltage/1(Upcc) -> "2nd-Order Filter  "/1
  "2nd-Order Filter  "/1 -> U_meas/1
  Active_Power/1(Ppcc) -> 2nd-Order Filter/1
  2nd-Order Filter/1 -> P_meas/1
  Reactive_Power/1(Qpcc) -> 2nd-Order Filter2/1
  2nd-Order Filter2/1 -> Q_meas/1
  Modulation_Index/1(Mod_index) -> "2nd-Order Filter "/1
  Demux/2 -> DC_Voltage/2(Udc_n)
  Uf_AB/1 -> Filter_Bus_Voltage/1(Uf_AB)
  U_AB/1 -> PCC_Voltage/1(U_AB), Active_Power/1(U_AB), Reactive_Power/1(U_AB)
  I_AB/1 -> Active_Power/2(I_AB), Reactive_Power/2(I_AB)
  DC_Voltage/1(Udc_meas) -> Product5/1, Udc_meas/1, Modulation_Index/2(Udc_meas)
  DC_Current/1(Idc_meas) -> Variable Frequency Mean value IC: 0/2
  Udc_pn/1 -> Demux/1
  Demux/1 -> DC_Voltage/1(Udc_p)
  Demux1/1 -> DC_Current/1(Idc_p)
  Demux1/2 -> DC_Current/2(Idc_n)
  Idc_pn/1 -> Demux1/1
  Vref_lim_AB/1 -> Modulation_Index/1(Vref_lim_AB)

== system HVDC_VSC_1CPUcore_dcpl/SM_HVDC_VSC/VSC Controller (Station 2)/Discrete VSC Controller (Station 2)/dq  Transformations ==
  note: dq Transformations
  U_AB : Inport
  Iv_AB : Inport  Port=2
  sin_cos : Inport  Port=3
  Constant1 : Constant  Value=0
  Mux1 : Mux  Inputs=[2 1]
  Mux4 : Mux  Inputs=[2 1]
  Selector : Selector  InputPortWidth=3  Indices=[1 2]
  Selector3 : Selector  InputPortWidth=3  Indices=[1 2]
  ab0_to_dq0 : Subsystem  AncestorBlock=lib_mesures/CLARK
  "ab0_to_dq0   " : Subsystem  AncestorBlock=lib_mesures/CLARK
  U_dq : Outport
  Iv_dq : Outport  Port=2
  wires:
  Constant1/1 -> Mux4/2, Mux1/2
  Mux4/1 -> "ab0_to_dq0   "/1(ab0)
  Iv_AB/1 -> Mux4/1
  Mux1/1 -> ab0_to_dq0/1(ab0)
  U_AB/1 -> Mux1/1
  "ab0_to_dq0   "/1(dq0) -> Selector3/1
  ab0_to_dq0/1(dq0) -> Selector/1
  sin_cos/1 -> "ab0_to_dq0   "/2(sin_cos), ab0_to_dq0/2(sin_cos)
  Selector/1 -> U_dq/1
  Selector3/1 -> Iv_dq/1

== system HVDC_VSC_1CPUcore_dcpl/SM_HVDC_VSC/WSCC System 1/Bus_4 230 KV/Three-Phase V-I Measurement1 ==
  Kv : Gain  Gain=Ki  SaturateOnIntegerOverflow=on  OutDataTypeStr=Inherit: Same as input  ParamDataTypeStr=Inherit: Same as input
  Kv1 : Gain  Gain=Kv  SaturateOnIntegerOverflow=on  OutDataTypeStr=Inherit: Same as input  ParamDataTypeStr=Inherit: Same as input
  Mode I : spsVIMeasurementModel/Complex
  Mode V : spsVIMeasurementModel/Complex
  Model : spsVIMeasurementModel/VI_phase  SystemSampleTime=-1
  A : PMIOPort  Port=1  Side=Left
  B : PMIOPort  Port=2  Side=Left
  C : PMIOPort  Port=3  Side=Left
  a : PMIOPort  Port=4  Side=Right
  b : PMIOPort  Port=5  Side=Right
  c : PMIOPort  Port=6  Side=Right
  tag scope: Iabc_45=global, Vabc_45=global
  wires:
  Model/2 -> Kv/1
  Model/1 -> Kv1/1
  Kv/1 -> Mode I/1
  Kv1/1 -> Mode V/1
  Mode I/1 -> [Iabc_45]
  Mode V/1 -> [Vabc_45]
  connections:
  Model/RConn3 -- c/RConn1
  Model/RConn1 -- a/RConn1
  Model/RConn2 -- b/RConn1
  Model/LConn3 -- C/RConn1
  Model/LConn1 -- A/RConn1
  Model/LConn2 -- B/RConn1

== system HVDC_VSC_1CPUcore_dcpl/SM_HVDC_VSC/WSCC System 1/Bus_4 230 KV/Three-Phase V-I Measurement3 ==
  Kv : Gain  Gain=Ki  SaturateOnIntegerOverflow=on  OutDataTypeStr=Inherit: Same as input  ParamDataTypeStr=Inherit: Same as input
  Kv1 : Gain  Gain=Kv  SaturateOnIntegerOverflow=on  OutDataTypeStr=Inherit: Same as input  ParamDataTypeStr=Inherit: Same as input
  Mode I : spsVIMeasurementModel/Complex
  Mode V : spsVIMeasurementModel/Complex
  Model : spsVIMeasurementModel/VI_phase  SystemSampleTime=-1
  A : PMIOPort  Port=1  Side=Left
  B : PMIOPort  Port=2  Side=Left
  C : PMIOPort  Port=3  Side=Left
  a : PMIOPort  Port=4  Side=Right
  b : PMIOPort  Port=5  Side=Right
  c : PMIOPort  Port=6  Side=Right
  tag scope: Iabc_46=global, Vabc_46=global
  wires:
  Model/2 -> Kv/1
  Model/1 -> Kv1/1
  Kv/1 -> Mode I/1
  Kv1/1 -> Mode V/1
  Mode I/1 -> [Iabc_46]
  Mode V/1 -> [Vabc_46]
  connections:
  Model/RConn3 -- c/RConn1
  Model/RConn1 -- a/RConn1
  Model/RConn2 -- b/RConn1
  Model/LConn3 -- C/RConn1
  Model/LConn1 -- A/RConn1
  Model/LConn2 -- B/RConn1

== system HVDC_VSC_1CPUcore_dcpl/SM_HVDC_VSC/WSCC System 1/Bus_7 230 KV/Three-Phase V-I Measurement1 ==
  Kv : Gain  Gain=Ki  SaturateOnIntegerOverflow=on  OutDataTypeStr=Inherit: Same as input  ParamDataTypeStr=Inherit: Same as input
  Kv1 : Gain  Gain=Kv  SaturateOnIntegerOverflow=on  OutDataTypeStr=Inherit: Same as input  ParamDataTypeStr=Inherit: Same as input
  Mode I : spsVIMeasurementModel/Complex
  Mode V : spsVIMeasurementModel/Complex
  Model : spsVIMeasurementModel/VI_phase  SystemSampleTime=-1
  A : PMIOPort  Port=1  Side=Left
  B : PMIOPort  Port=2  Side=Left
  C : PMIOPort  Port=3  Side=Left
  a : PMIOPort  Port=4  Side=Right
  b : PMIOPort  Port=5  Side=Right
  c : PMIOPort  Port=6  Side=Right
  tag scope: Iabc_7=global, Vabc_7=global
  wires:
  Model/2 -> Kv/1
  Model/1 -> Kv1/1
  Kv/1 -> Mode I/1
  Kv1/1 -> Mode V/1
  Mode I/1 -> [Iabc_7]
  Mode V/1 -> [Vabc_7]
  connections:
  Model/RConn3 -- c/RConn1
  Model/RConn1 -- a/RConn1
  Model/RConn2 -- b/RConn1
  Model/LConn3 -- C/RConn1
  Model/LConn1 -- A/RConn1
  Model/LConn2 -- B/RConn1

== system HVDC_VSC_1CPUcore_dcpl/SM_HVDC_VSC/WSCC System 1/Bus_7 230 KV/Three-Phase V-I Measurement3 ==
  Kv : Gain  Gain=Ki  SaturateOnIntegerOverflow=on  OutDataTypeStr=Inherit: Same as input  ParamDataTypeStr=Inherit: Same as input
  Kv1 : Gain  Gain=Kv  SaturateOnIntegerOverflow=on  OutDataTypeStr=Inherit: Same as input  ParamDataTypeStr=Inherit: Same as input
  Mode I : spsVIMeasurementModel/Complex
  Mode V : spsVIMeasurementModel/Complex
  Model : spsVIMeasurementModel/VI_phase  SystemSampleTime=-1
  A : PMIOPort  Port=1  Side=Left
  B : PMIOPort  Port=2  Side=Left
  C : PMIOPort  Port=3  Side=Left
  a : PMIOPort  Port=4  Side=Right
  b : PMIOPort  Port=5  Side=Right
  c : PMIOPort  Port=6  Side=Right
  tag scope: Iab=global, Vabc=global
  wires:
  Model/2 -> Kv/1
  Model/1 -> Kv1/1
  Kv/1 -> Mode I/1
  Kv1/1 -> Mode V/1
  Mode I/1 -> [Iab]
  Mode V/1 -> [Vabc]
  connections:
  Model/RConn3 -- c/RConn1
  Model/RConn1 -- a/RConn1
  Model/RConn2 -- b/RConn1
  Model/LConn3 -- C/RConn1
  Model/LConn1 -- A/RConn1
  Model/LConn2 -- B/RConn1

== system HVDC_VSC_1CPUcore_dcpl/SM_HVDC_VSC/WSCC System 1/Bus_9 230 KV/Three-Phase V-I Measurement1 ==
  Kv : Gain  Gain=Ki  SaturateOnIntegerOverflow=on  OutDataTypeStr=Inherit: Same as input  ParamDataTypeStr=Inherit: Same as input
  Kv1 : Gain  Gain=Kv  SaturateOnIntegerOverflow=on  OutDataTypeStr=Inherit: Same as input  ParamDataTypeStr=Inherit: Same as input
  Mode I : spsVIMeasurementModel/Complex
  Mode V : spsVIMeasurementModel/Complex
  Model : spsVIMeasurementModel/VI_phase  SystemSampleTime=-1
  A : PMIOPort  Port=1  Side=Left
  B : PMIOPort  Port=2  Side=Left
  C : PMIOPort  Port=3  Side=Left
  a : PMIOPort  Port=4  Side=Right
  b : PMIOPort  Port=5  Side=Right
  c : PMIOPort  Port=6  Side=Right
  tag scope: Iabc_9=global, Vabc_9=global
  wires:
  Model/2 -> Kv/1
  Model/1 -> Kv1/1
  Kv/1 -> Mode I/1
  Kv1/1 -> Mode V/1
  Mode I/1 -> [Iabc_9]
  Mode V/1 -> [Vabc_9]
  connections:
  Model/RConn3 -- c/RConn1
  Model/RConn1 -- a/RConn1
  Model/RConn2 -- b/RConn1
  Model/LConn3 -- C/RConn1
  Model/LConn1 -- A/RConn1
  Model/LConn2 -- B/RConn1

== system HVDC_VSC_1CPUcore_dcpl/SM_HVDC_VSC/WSCC System 1/Bus_9 230 KV/Three-Phase V-I Measurement3 ==
  Kv : Gain  Gain=Ki  SaturateOnIntegerOverflow=on  OutDataTypeStr=Inherit: Same as input  ParamDataTypeStr=Inherit: Same as input
  Kv1 : Gain  Gain=Kv  SaturateOnIntegerOverflow=on  OutDataTypeStr=Inherit: Same as input  ParamDataTypeStr=Inherit: Same as input
  Mode I : spsVIMeasurementModel/Complex
  Mode V : spsVIMeasurementModel/Complex
  Model : spsVIMeasurementModel/VI_phase  SystemSampleTime=-1
  A : PMIOPort  Port=1  Side=Left
  B : PMIOPort  Port=2  Side=Left
  C : PMIOPort  Port=3  Side=Left
  a : PMIOPort  Port=4  Side=Right
  b : PMIOPort  Port=5  Side=Right
  c : PMIOPort  Port=6  Side=Right
  tag scope: Iabc_10=global, Vabc_10=global
  wires:
  Model/2 -> Kv/1
  Model/1 -> Kv1/1
  Kv/1 -> Mode I/1
  Kv1/1 -> Mode V/1
  Mode I/1 -> [Iabc_10]
  Mode V/1 -> [Vabc_10]
  connections:
  Model/RConn3 -- c/RConn1
  Model/RConn1 -- a/RConn1
  Model/RConn2 -- b/RConn1
  Model/LConn3 -- C/RConn1
  Model/LConn1 -- A/RConn1
  Model/LConn2 -- B/RConn1

== system HVDC_VSC_1CPUcore_dcpl/SM_HVDC_VSC/WSCC System 1/Generator BUS1x1/Subsystem1 ==
  In1 : Inport
  In2 : Inport  Port=2
  In3 : Inport  Port=3
  Gain : Gain  Gain=-1  SaturateOnIntegerOverflow=on  OutDataTypeStr=Inherit: Same as input  ParamDataTypeStr=Inherit: Same as input
  Mux : Mux  Inputs=2
  Selector : Selector  InputPortWidth=4  Indices=[4 3]
  Selector1 : Selector  InputPortWidth=4  Indices=[4 3]
  dw_123 : Outport
  T_23 : Outport  Port=2
  wires:
  Selector/1 -> Mux/2
  Mux/1 -> dw_123/1
  In1/1 -> Mux/1
  In2/1 -> Selector/1
  In3/1 -> Selector1/1
  Selector1/1 -> Gain/1
  Gain/1 -> T_23/1

== system HVDC_VSC_1CPUcore_dcpl/SM_HVDC_VSC/WSCC System 1/Generator BUS2x1/Subsystem1 ==
  In1 : Inport
  In2 : Inport  Port=2
  In3 : Inport  Port=3
  Gain : Gain  Gain=-1  SaturateOnIntegerOverflow=on  OutDataTypeStr=Inherit: Same as input  ParamDataTypeStr=Inherit: Same as input
  Mux : Mux  Inputs=2
  Selector : Selector  InputPortWidth=4  Indices=[4 3]
  Selector1 : Selector  InputPortWidth=4  Indices=[4 3]
  dw_123 : Outport
  T_23 : Outport  Port=2
  wires:
  Selector/1 -> Mux/2
  Mux/1 -> dw_123/1
  In1/1 -> Mux/1
  In2/1 -> Selector/1
  In3/1 -> Selector1/1
  Selector1/1 -> Gain/1
  Gain/1 -> T_23/1

== system HVDC_VSC_1CPUcore_dcpl/SM_HVDC_VSC/WSCC System 1/Generator BUS3x1/Subsystem1 ==
  In1 : Inport
  In2 : Inport  Port=2
  In3 : Inport  Port=3
  Gain : Gain  Gain=-1  SaturateOnIntegerOverflow=on  OutDataTypeStr=Inherit: Same as input  ParamDataTypeStr=Inherit: Same as input
  Mux : Mux  Inputs=2
  Selector : Selector  InputPortWidth=4  Indices=[4 3]
  Selector1 : Selector  InputPortWidth=4  Indices=[4 3]
  dw_123 : Outport
  T_23 : Outport  Port=2
  wires:
  Selector/1 -> Mux/2
  Mux/1 -> dw_123/1
  In1/1 -> Mux/1
  In2/1 -> Selector/1
  In3/1 -> Selector1/1
  Selector1/1 -> Gain/1
  Gain/1 -> T_23/1

== system HVDC_VSC_1CPUcore_dcpl/SM_HVDC_VSC/WSCC System 2/Bus_4 230 KV/Three-Phase V-I Measurement1 ==
  Kv : Gain  Gain=Ki  SaturateOnIntegerOverflow=on  OutDataTypeStr=Inherit: Same as input  ParamDataTypeStr=Inherit: Same as input
  Kv1 : Gain  Gain=Kv  SaturateOnIntegerOverflow=on  OutDataTypeStr=Inherit: Same as input  ParamDataTypeStr=Inherit: Same as input
  Mode I : spsVIMeasurementModel/Complex
  Mode V : spsVIMeasurementModel/Complex
  Model : spsVIMeasurementModel/VI_phase  SystemSampleTime=-1
  A : PMIOPort  Port=1  Side=Left
  B : PMIOPort  Port=2  Side=Left
  C : PMIOPort  Port=3  Side=Left
  a : PMIOPort  Port=4  Side=Right
  b : PMIOPort  Port=5  Side=Right
  c : PMIOPort  Port=6  Side=Right
  tag scope: Iabc_245=global, Vabc_245=global
  wires:
  Model/2 -> Kv/1
  Model/1 -> Kv1/1
  Kv/1 -> Mode I/1
  Kv1/1 -> Mode V/1
  Mode I/1 -> [Iabc_245]
  Mode V/1 -> [Vabc_245]
  connections:
  Model/RConn3 -- c/RConn1
  Model/RConn1 -- a/RConn1
  Model/RConn2 -- b/RConn1
  Model/LConn3 -- C/RConn1
  Model/LConn1 -- A/RConn1
  Model/LConn2 -- B/RConn1

== system HVDC_VSC_1CPUcore_dcpl/SM_HVDC_VSC/WSCC System 2/Bus_4 230 KV/Three-Phase V-I Measurement3 ==
  Kv : Gain  Gain=Ki  SaturateOnIntegerOverflow=on  OutDataTypeStr=Inherit: Same as input  ParamDataTypeStr=Inherit: Same as input
  Kv1 : Gain  Gain=Kv  SaturateOnIntegerOverflow=on  OutDataTypeStr=Inherit: Same as input  ParamDataTypeStr=Inherit: Same as input
  Mode I : spsVIMeasurementModel/Complex
  Mode V : spsVIMeasurementModel/Complex
  Model : spsVIMeasurementModel/VI_phase  SystemSampleTime=-1
  A : PMIOPort  Port=1  Side=Left
  B : PMIOPort  Port=2  Side=Left
  C : PMIOPort  Port=3  Side=Left
  a : PMIOPort  Port=4  Side=Right
  b : PMIOPort  Port=5  Side=Right
  c : PMIOPort  Port=6  Side=Right
  tag scope: Iabc_246=global, Vabc_246=global
  wires:
  Model/2 -> Kv/1
  Model/1 -> Kv1/1
  Kv/1 -> Mode I/1
  Kv1/1 -> Mode V/1
  Mode I/1 -> [Iabc_246]
  Mode V/1 -> [Vabc_246]
  connections:
  Model/RConn3 -- c/RConn1
  Model/RConn1 -- a/RConn1
  Model/RConn2 -- b/RConn1
  Model/LConn3 -- C/RConn1
  Model/LConn1 -- A/RConn1
  Model/LConn2 -- B/RConn1

== system HVDC_VSC_1CPUcore_dcpl/SM_HVDC_VSC/WSCC System 2/Bus_7 230 KV/Three-Phase V-I Measurement1 ==
  Kv : Gain  Gain=Ki  SaturateOnIntegerOverflow=on  OutDataTypeStr=Inherit: Same as input  ParamDataTypeStr=Inherit: Same as input
  Kv1 : Gain  Gain=Kv  SaturateOnIntegerOverflow=on  OutDataTypeStr=Inherit: Same as input  ParamDataTypeStr=Inherit: Same as input
  Mode I : spsVIMeasurementModel/Complex
  Mode V : spsVIMeasurementModel/Complex
  Model : spsVIMeasurementModel/VI_phase  SystemSampleTime=-1
  A : PMIOPort  Port=1  Side=Left
  B : PMIOPort  Port=2  Side=Left
  C : PMIOPort  Port=3  Side=Left
  a : PMIOPort  Port=4  Side=Right
  b : PMIOPort  Port=5  Side=Right
  c : PMIOPort  Port=6  Side=Right
  tag scope: Iabc_27=global, Vabc_27=global
  wires:
  Model/2 -> Kv/1
  Model/1 -> Kv1/1
  Kv/1 -> Mode I/1
  Kv1/1 -> Mode V/1
  Mode I/1 -> [Iabc_27]
  Mode V/1 -> [Vabc_27]
  connections:
  Model/RConn3 -- c/RConn1
  Model/RConn1 -- a/RConn1
  Model/RConn2 -- b/RConn1
  Model/LConn3 -- C/RConn1
  Model/LConn1 -- A/RConn1
  Model/LConn2 -- B/RConn1

== system HVDC_VSC_1CPUcore_dcpl/SM_HVDC_VSC/WSCC System 2/Bus_7 230 KV/Three-Phase V-I Measurement3 ==
  Kv : Gain  Gain=Ki  SaturateOnIntegerOverflow=on  OutDataTypeStr=Inherit: Same as input  ParamDataTypeStr=Inherit: Same as input
  Kv1 : Gain  Gain=Kv  SaturateOnIntegerOverflow=on  OutDataTypeStr=Inherit: Same as input  ParamDataTypeStr=Inherit: Same as input
  Mode I : spsVIMeasurementModel/Complex
  Mode V : spsVIMeasurementModel/Complex
  Model : spsVIMeasurementModel/VI_phase  SystemSampleTime=-1
  A : PMIOPort  Port=1  Side=Left
  B : PMIOPort  Port=2  Side=Left
  C : PMIOPort  Port=3  Side=Left
  a : PMIOPort  Port=4  Side=Right
  b : PMIOPort  Port=5  Side=Right
  c : PMIOPort  Port=6  Side=Right
  tag scope: Iab_20=global, Vabc_20=global
  wires:
  Model/2 -> Kv/1
  Model/1 -> Kv1/1
  Kv/1 -> Mode I/1
  Kv1/1 -> Mode V/1
  Mode I/1 -> [Iab_20]
  Mode V/1 -> [Vabc_20]
  connections:
  Model/RConn3 -- c/RConn1
  Model/RConn1 -- a/RConn1
  Model/RConn2 -- b/RConn1
  Model/LConn3 -- C/RConn1
  Model/LConn1 -- A/RConn1
  Model/LConn2 -- B/RConn1

== system HVDC_VSC_1CPUcore_dcpl/SM_HVDC_VSC/WSCC System 2/Bus_9 230 KV/Three-Phase V-I Measurement1 ==
  Kv : Gain  Gain=Ki  SaturateOnIntegerOverflow=on  OutDataTypeStr=Inherit: Same as input  ParamDataTypeStr=Inherit: Same as input
  Kv1 : Gain  Gain=Kv  SaturateOnIntegerOverflow=on  OutDataTypeStr=Inherit: Same as input  ParamDataTypeStr=Inherit: Same as input
  Mode I : spsVIMeasurementModel/Complex
  Mode V : spsVIMeasurementModel/Complex
  Model : spsVIMeasurementModel/VI_phase  SystemSampleTime=-1
  A : PMIOPort  Port=1  Side=Left
  B : PMIOPort  Port=2  Side=Left
  C : PMIOPort  Port=3  Side=Left
  a : PMIOPort  Port=4  Side=Right
  b : PMIOPort  Port=5  Side=Right
  c : PMIOPort  Port=6  Side=Right
  tag scope: Iabc_29=global, Vabc_29=global
  wires:
  Model/2 -> Kv/1
  Model/1 -> Kv1/1
  Kv/1 -> Mode I/1
  Kv1/1 -> Mode V/1
  Mode I/1 -> [Iabc_29]
  Mode V/1 -> [Vabc_29]
  connections:
  Model/RConn3 -- c/RConn1
  Model/RConn1 -- a/RConn1
  Model/RConn2 -- b/RConn1
  Model/LConn3 -- C/RConn1
  Model/LConn1 -- A/RConn1
  Model/LConn2 -- B/RConn1
